simulink library "passive_model"  (R2018a)
settings: Solver=VariableStepAuto  StartTime=0.0  StopTime=10.0  RelTol=1e-3
values from neighbouring files (symbols this model uses):
  c = 1000    [parameters.m]
  k = 16812    [parameters.m]
  kt = 190000    [parameters.m]
  ms = 105    [parameters.m]
  mu = 50    [parameters.m]
settings Model: Creator=Saurabh Suman  LastModifiedBy=Saurabh Suman

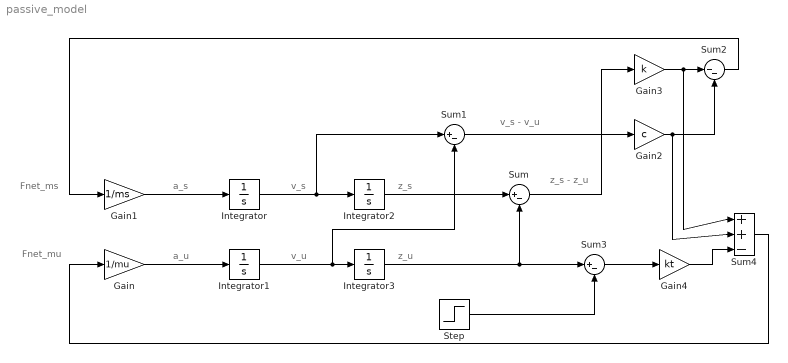
== system passive_model ==
  note: z_s - z_u
  note: v_s - v_u
  note: Fnet_mu
  note: Fnet_ms
  note: a_u
  note: z_u
  note: z_s
  note: a_s
  note: v_s
  note: v_u
  Gain : Gain  Gain=1/mu
  Gain1 : Gain  Gain=1/ms
  Gain2 : Gain  Gain=c
  Gain3 : Gain  Gain=k
  Gain4 : Gain  Gain=kt
  Integrator{,1..3} (4 alike) : Integrator
  Step : Step  SampleTime=0
  Sum : Sum  Inputs=|+-
  Sum1 : Sum  Inputs=|+-
  Sum2 : Sum  Inputs=|--
  Sum3 : Sum  Inputs=|+-
  Sum4 : Sum  Inputs=|++-
  wires:
  Integrator/1 -> Sum1/1, Integrator2/1
  Integrator1/1 -> Sum1/2, Integrator3/1
  Integrator2/1 -> Sum/1
  Gain1/1 -> Integrator/1
  Gain/1 -> Integrator1/1
  Integrator3/1 -> Sum3/1, Sum/2
  Sum2/1 -> Gain1/1
  Sum4/1 -> Gain/1
  Sum1/1 -> Gain2/1
  Sum/1 -> Gain3/1
  Gain3/1 -> Sum4/1, Sum2/1
  Gain2/1 -> Sum4/2, Sum2/2
  Step/1 -> Sum3/2
  Sum3/1 -> Gain4/1
  Gain4/1 -> Sum4/3
